simulink model "onduleursimplecommande"  (Simulink 7.9)
settings: Solver=VariableStepDiscrete  StartTime=0.0  StopTime=0.2  RelTol=1e-3
libraries: powerlib x20, powerlib_extras x3
settings Model: Creator=LiberT  LastModifiedBy=LiberT

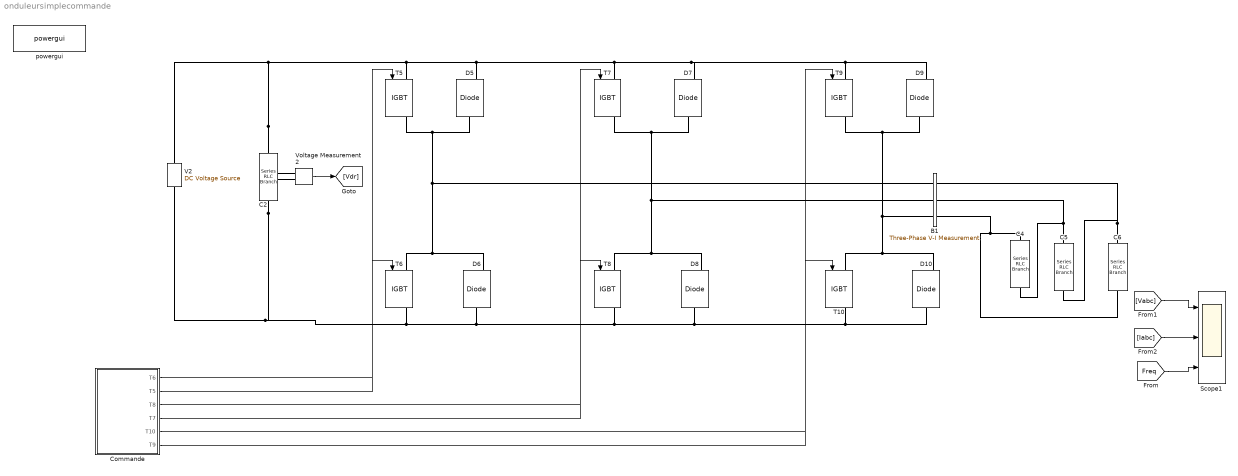
== system onduleursimplecommande ==
  B1 : powerlib/Measurements/Three-Phase V-I Measurement  VoltageMeasurement=phase-to-phase  SetLabelV=on  LabelV=Vabc  Vpu=off  VpuLL=off  CurrentMeasurement=yes  SetLabelI=on  LabelI=Iabc  Ipu=off  Pbase=100e6  Vbase=500e3  OutputType=Complex  PhasorSimulation=off  PSBequivalent=0
  C2 : powerlib/Elements/Series RLC Branch  LConnTagsString=__new0  RConnTagsString=__new0  BranchType=Open circuit  Resistance=0.28  Inductance=1e-3  SetiL0=off  InitialCurrent=0  Capacitance=300e-1  Setx0=off  InitialVoltage=0  Measurements=None
  C4 : powerlib/Elements/Series RLC Branch  LConnTagsString=__new0  RConnTagsString=__new0  BranchType=RL  Resistance=0.28  Inductance=0.005  SetiL0=off  InitialCurrent=0  Capacitance=300e-3  Setx0=off  InitialVoltage=0  Measurements=None
  C5 : powerlib/Elements/Series RLC Branch  LConnTagsString=__new0  RConnTagsString=__new0  BranchType=RL  Resistance=0.28  Inductance=0.005  SetiL0=off  InitialCurrent=0  Capacitance=300e-3  Setx0=off  InitialVoltage=0  Measurements=None
  C6 : powerlib/Elements/Series RLC Branch  LConnTagsString=__new0  RConnTagsString=__new0  BranchType=RL  Resistance=0.28  Inductance=0.005  SetiL0=off  InitialCurrent=0  Capacitance=300e-3  Setx0=off  InitialVoltage=0  Measurements=None
  Commande : Subsystem  mask{Iac=40, Fac=50}
      mask prompts: Iac "Maximum de courant (A)"; Fac "Fréquence (Hz)"
  D{5..10} (6 alike) : powerlib/Power Electronics/Diode  Ron=0.001  Lon=0  Vf=0.8  IC=0  UseSnubber=off  Rs=500  Cs=250e-9  Measurements=on
  Scope1 : Scope  NumInputPorts=3
      settings: YMin=-125~-45~49.525  YMax=125~45~50.05
  T{5..10} (6 alike) : powerlib/Power Electronics/IGBT  Ron=0.001  Lon=0  Vf=1  Tf=1e-6  Tt=2e-6  IC=0  Rs=1e5  Cs=inf  Measurements=on
  V2 : powerlib/Electrical Sources/DC Voltage Source  Amplitude=100  Measurements=None
  Voltage Measurement2 : powerlib/Measurements/Voltage Measurement  PhasorSimulation=off  OutputType=Complex  PSBequivalent=0
  powergui : powerlib/powergui  Priority=1  SimulationMode=Discrete  SolverType=Tustin  SampleTime=50e-7  frequency=60  SPID=off  DisableSnubberDevices=off  DisableRonSwitches=off  DisableVfSwitches=off  SwTol=0  Interpol=off  DisplayEquations=off  FunctionMessages=off  frequencyindice=0  Pbase=100e6  ErrMax=1e-4  Iterations=50  UnitsV=kV  UnitsW=MW  echomessages=off  HookPort=off  EnableUseOfTLC=off  x0status=blocks  RestoreLinks=warning  ResistiveCurrentMeasurement=off  Ylog=off  Xlog=on  ShowGrid=off  save=off  variable=ZData  ZoomFFT=off  StartTime=0.0  cycles=1  DisplayStyle=1  FreqAxis=off  MaxFrequency=1000  frequencyindicesteady=1  display=off  methode=off
  wires:
  Voltage Measurement2/1 -> [Vdr]
  [Freq] -> Scope1/3
  Commande/6(T9) -> T9/1
  Commande/5(T10) -> T10/1
  Commande/4(T7) -> T7/1
  Commande/3(T8) -> T8/1
  [Vabc] -> Scope1/1
  [Iabc] -> Scope1/2
  Commande/2(T5) -> T5/1
  Commande/1(T6) -> T6/1
  connections:
  C2/RConn1 -- V2/LConn1 -- T6/RConn1 -- D6/LConn1 -- T8/RConn1 -- D8/LConn1 -- T10/RConn1 -- D10/LConn1 -- Voltage Measurement2/LConn2
  C6/LConn1 -- B1/RConn1 -- C5/RConn1
  B1/RConn2 -- C5/LConn1 -- C4/RConn1
  T9/RConn1 -- D9/LConn1 -- T10/LConn1 -- D10/RConn1 -- B1/LConn3
  B1/RConn3 -- C4/LConn1 -- C6/RConn1
  C2/LConn1 -- Voltage Measurement2/LConn1 -- T5/LConn1 -- D5/RConn1 -- T7/LConn1 -- D7/RConn1 -- T9/LConn1 -- D9/RConn1 -- V2/RConn1
  T8/LConn1 -- D8/RConn1 -- T7/RConn1 -- D7/LConn1 -- B1/LConn2
  T5/RConn1 -- D5/LConn1 -- T6/LConn1 -- D6/RConn1 -- B1/LConn1

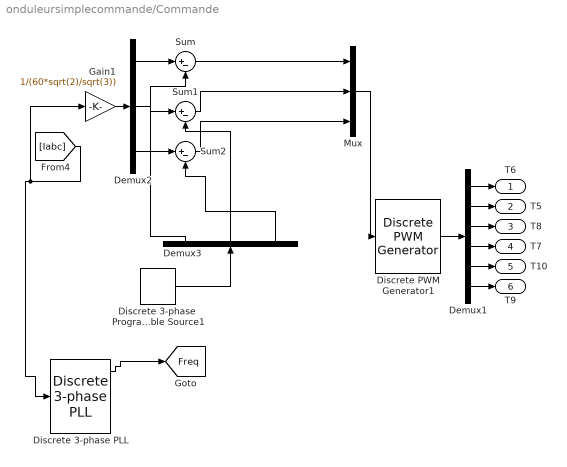
== system onduleursimplecommande/Commande ==
  Demux1 : Demux  Outputs=6
  Demux2 : Demux  Outputs=3
  Demux3 : Demux  Outputs=3
  Discrete 3-phase  Programmable Source1 : powerlib_extras/Discrete  Control Blocks/Discrete 3-phase  Programmable Source  Par_Vps=[Iac/40 90 Fac]  VariationEntity=None  VariationType=Step  VariationStep=-0.5  VariationRate=10  VariationMag=0.3  VariationFreq=2  Par_Timing_Variation=[0.1 1.2]  SinglePhase=on  Yampli=[1 0.2 1.2 1.0]  Xtime=[0 0.1 0.15 0.2]  HarmonicGeneration=off  Par_HarmoA=[3 0.2 -25 0]  Par_HarmoB=[2 0.15 35 2]  Par_Timing_Harmo="[0.05  3]"  Ts=5e-6
  Discrete 3-phase PLL : powerlib_extras/Discrete  Control Blocks/Discrete 3-phase PLL  Fmin=45  Par_Init=[0 50]  ParK=[ 180 3200 1 ]  Ts=50e-6  AGC=off
  Discrete PWM Generator1 : powerlib_extras/Discrete  Control Blocks/Discrete PWM Generator  GeneratorMode="3-arm  bridge (6 pulses)"  Fc=1000  Ts=5e-6  Internal=off  mIndex=1  Freq=60  Phase=0
  Gain1 : Gain  Gain=1/(60*sqrt(2)/sqrt(3))
  Mux : Mux  Inputs=3
  Sum : Sum  Inputs=|+-
  Sum1 : Sum  Inputs=|+-
  Sum2 : Sum  Inputs=|+-
  T6 : Outport
  T5 : Outport  Port=2
  T8 : Outport  Port=3
  T7 : Outport  Port=4
  T10 : Outport  Port=5
  T9 : Outport  Port=6
  tag scope: Freq=global
  wires:
  Discrete PWM Generator1/1 -> Demux1/1
  Demux2/1 -> Sum/1
  Demux3/1 -> Sum/2
  Demux2/2 -> Sum1/1
  Demux2/3 -> Sum2/1
  Demux3/2 -> Sum1/2
  Demux3/3 -> Sum2/2
  [Iabc] -> Gain1/1, Discrete 3-phase PLL/1
  Gain1/1 -> Demux2/1
  Discrete 3-phase  Programmable Source1/1 -> Demux3/1
  Sum/1 -> Mux/1
  Sum1/1 -> Mux/2
  Sum2/1 -> Mux/3
  Mux/1 -> Discrete PWM Generator1/1
  Demux1/1 -> T6/1
  Demux1/3 -> T8/1
  Demux1/4 -> T7/1
  Demux1/5 -> T10/1
  Demux1/6 -> T9/1
  Demux1/2 -> T5/1
  Discrete 3-phase PLL/1 -> [Freq]
